simulink model "Electrical"  (R2021a)
settings: Solver=VariableStepAuto  StartTime=0.0  StopTime=10.0  RelTol=1e-3
values from neighbouring files (symbols this model uses):
  Jeq = Jm+Jh+Jp    (= 1.120304e-05)    [QuanserData.m]
  k1 = 1.2e-5    (= 1.2e-05)    [QuanserData.m]
  k2 = 3.54e-9    (= 3.54e-09)    [QuanserData.m]
  k3 = -9.06e-5    (= -9.06e-05)    [QuanserData.m]
  k4 = 7.83e-7    (= 7.83e-07)    [QuanserData.m]
  km = 0.042    [QuanserData.m]
  Lm = 1.16e-3    (= 0.00116)    [QuanserData.m]
  Rm = 8.4    [QuanserData.m]
settings Model: Creator=y.briere  LastModifiedBy=fades
settings SolverCC: AlgebraicLoopSolver=TrustRegion
settings DataIOCC: ExternalInput=[0 15]  InitialState=[]  ReturnWorkspaceOutputs=off
settings OptimizationCC: DefaultParameterBehavior=Inlined  BufferReuse=off
settings DebuggingCC: InitInArrayFormatMsg=none  SFMachineParentedDataDiag=warning  ArithmeticOperatorsInVariantConditions=warning
settings SFSimCC: CustomCodeUndefinedFunction=UseInterfaceOnly

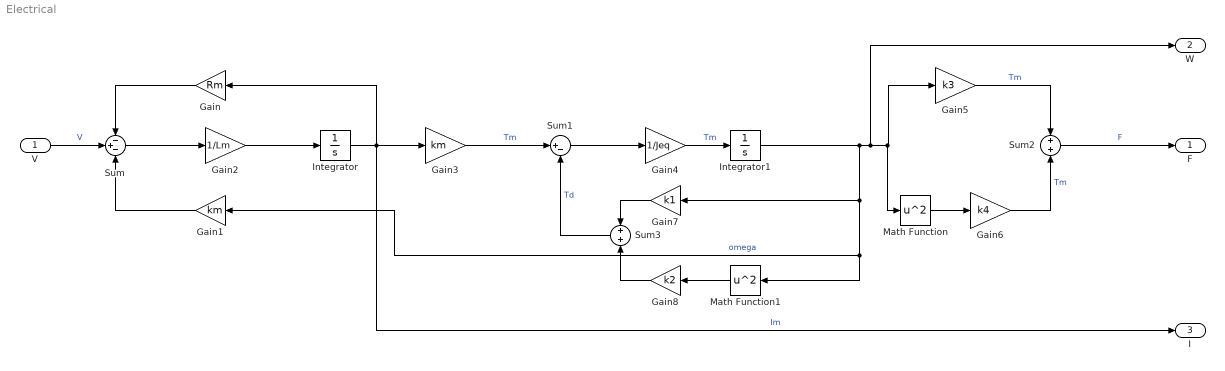
== system Electrical ==
  V : Inport
  Gain : Gain  Gain=Rm
  Gain1 : Gain  Gain=km
  Gain2 : Gain  Gain=1/Lm
  Gain3 : Gain  Gain=km
  Gain4 : Gain  Gain=1/Jeq
  Gain5 : Gain  Gain=k3
  Gain6 : Gain  Gain=k4
  Gain7 : Gain  Gain=k1
  Gain8 : Gain  Gain=k2
  Integrator : Integrator
  Integrator1 : Integrator
  Math Function : Math  Operator=square  SaturateOnIntegerOverflow=on
  Math Function1 : Math  Operator=square  SaturateOnIntegerOverflow=on
  Sum : Sum  Inputs=-+-
  Sum1 : Sum  Inputs=|+-
  Sum2 : Sum
  Sum3 : Sum
  F : Outport  VectorParamsAs1DForOutWhenUnconnected=off
  W : Outport  Port=2  VectorParamsAs1DForOutWhenUnconnected=off
  I : Outport  Port=3  VectorParamsAs1DForOutWhenUnconnected=off
  wires:
  V/1 -> Sum/2  "V"
  Sum2/1 -> F/1  "F"
  Gain/1 -> Sum/1
  Gain1/1 -> Sum/3
  Sum/1 -> Gain2/1
  Gain2/1 -> Integrator/1
  Integrator/1 -> I/1, Gain3/1, Gain/1  "Im"
  Gain3/1 -> Sum1/1  "Tm"
  Sum1/1 -> Gain4/1
  Gain4/1 -> Integrator1/1  "Tm"
  Integrator1/1 -> Math Function1/1, Gain1/1, Gain7/1, W/1, Math Function/1, Gain5/1  "omega"
  Math Function/1 -> Gain6/1
  Gain5/1 -> Sum2/1  "Tm"
  Gain6/1 -> Sum2/2  "Tm"
  Math Function1/1 -> Gain8/1
  Gain8/1 -> Sum3/2
  Gain7/1 -> Sum3/1
  Sum3/1 -> Sum1/2  "Td"
